simulink model "ex_1"  (R2023a)
settings: Solver=FixedStepAuto  StartTime=0.0  StopTime=10  FixedStep=1e-4  RelTol=1e-3
InitFcn:
  | Ki = 50;
  | Kd = 0;
  | Kp = 30;
settings Model: Creator=LabCom  LastModifiedBy=LabCom

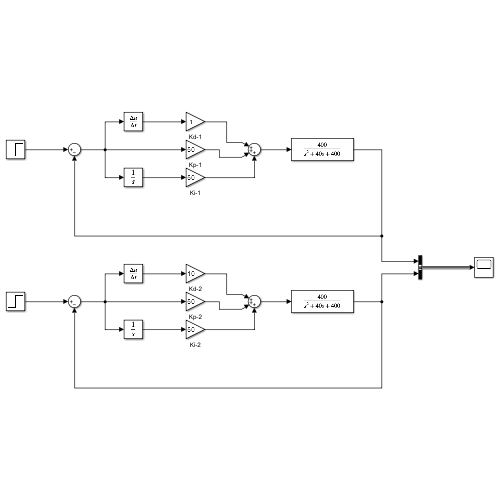
[thumbnail: Simulink's stored preview of the top-level diagram]
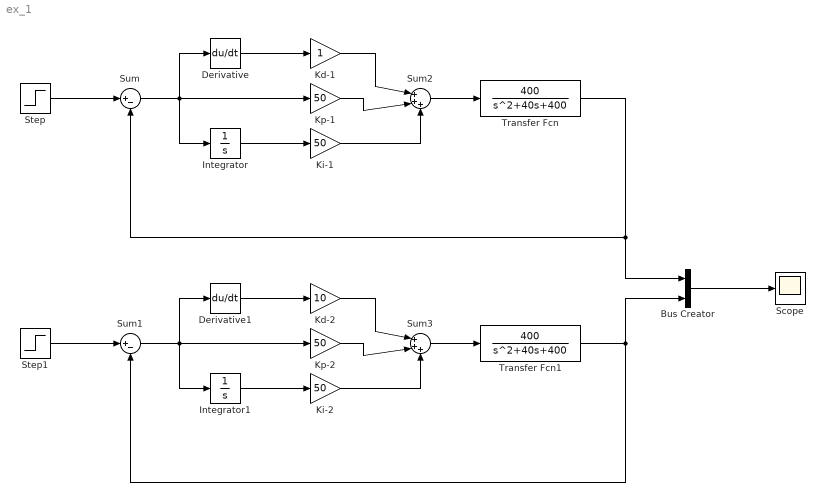
== system ex_1 ==
  Bus Creator : BusCreator  Inputs=2
  Derivative : Derivative
  Derivative1 : Derivative
  Integrator : Integrator
  Integrator1 : Integrator
  Kd-1 : Gain
  Kd-2 : Gain  Gain=10
  Ki-1 : Gain  Gain=50
  Ki-2 : Gain  Gain=50
  Kp-1 : Gain  Gain=50
  Kp-2 : Gain  Gain=50
  Scope : Scope
  Step : Step  Time=0  SampleTime=0
  Step1 : Step  Time=0  SampleTime=0
  Sum : Sum  Inputs=|+-
  Sum1 : Sum  Inputs=|+-
  Sum2 : Sum  Inputs=|+++
  Sum3 : Sum  Inputs=|+++
  Transfer Fcn : TransferFcn  Numerator=[400]  Denominator=[1 40 400]
  Transfer Fcn1 : TransferFcn  Numerator=[400]  Denominator=[1 40 400]
  wires:
  Derivative/1 -> Kd-1/1
  Kp-1/1 -> Sum2/2
  Sum/1 -> Integrator/1, Derivative/1, Kp-1/1
  Integrator/1 -> Ki-1/1
  Ki-1/1 -> Sum2/3
  Kd-1/1 -> Sum2/1
  Step/1 -> Sum/1
  Sum2/1 -> Transfer Fcn/1
  Transfer Fcn/1 -> Bus Creator/1, Sum/2
  Step1/1 -> Sum1/1
  Derivative1/1 -> Kd-2/1
  Ki-2/1 -> Sum3/3
  Sum3/1 -> Transfer Fcn1/1
  Transfer Fcn1/1 -> Bus Creator/2, Sum1/2
  Kd-2/1 -> Sum3/1
  Integrator1/1 -> Ki-2/1
  Kp-2/1 -> Sum3/2
  Sum1/1 -> Integrator1/1, Derivative1/1, Kp-2/1
  Bus Creator/1 -> Scope/1
